simulink model "detector"  (R2018b)
settings: Solver=FixedStepDiscrete  StartTime=0.0  StopTime=10.0  RelTol=1e-3
libraries: hdlsllib x18, simulink x18
settings Model: Creator=jayakumarav  LastModifiedBy=hiterd
settings DebuggingCC: LibraryContextMissingDiagnostic=none
settings SFSimCC: SimUseLocalCustomCode=off
settings RTWCC: RTWUseLocalCustomCode=off

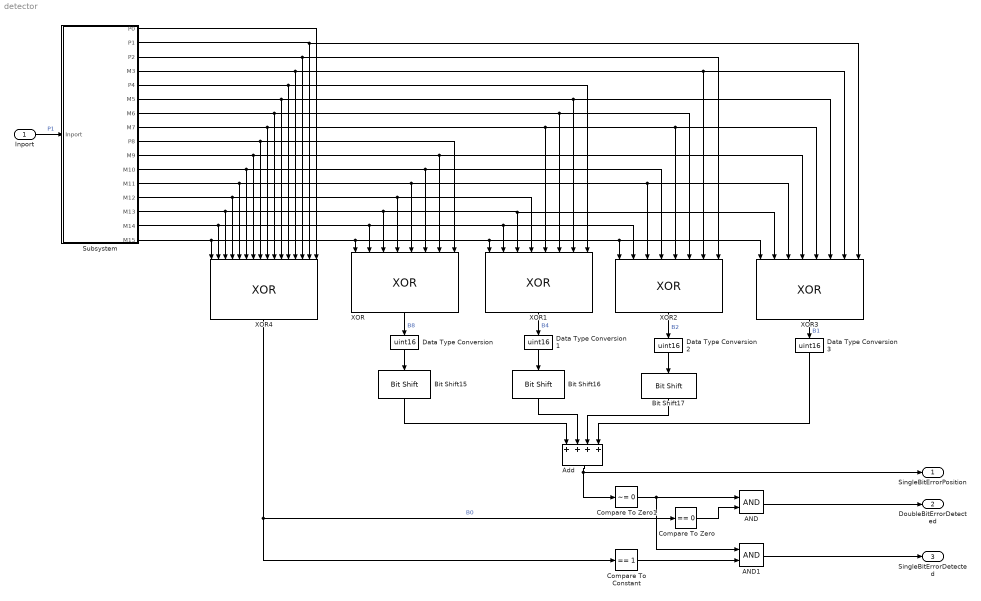
== system detector ==
  Inport : Inport
  AND : Logic  AllPortsSameDT=off  OutDataTypeStr=boolean
  AND1 : Logic  AllPortsSameDT=off  OutDataTypeStr=boolean
  Add : Sum  Inputs=++++
  Bit Shift15 : hdlsllib/Logic and Bit Operations/Bit Shift  mode=Shift Left Logical  N=3
      settings: SourceProductName=HDL Coder  SourceProductBaseCode=HD
  Bit Shift16 : hdlsllib/Logic and Bit Operations/Bit Shift  mode=Shift Left Logical  N=2
      settings: SourceProductName=HDL Coder  SourceProductBaseCode=HD
  Bit Shift17 : hdlsllib/Logic and Bit Operations/Bit Shift  mode=Shift Left Logical  N=1
      settings: SourceProductName=HDL Coder  SourceProductBaseCode=HD
  Compare To Constant : simulink/Logic and Bit Operations/Compare To Constant  relop===  const=1  OutDataTypeStr=boolean
  Compare To Zero : simulink/Logic and Bit Operations/Compare To Zero  relop===  OutDataTypeStr=boolean
  Compare To Zero1 : simulink/Logic and Bit Operations/Compare To Zero  relop=~=  OutDataTypeStr=boolean
  Data Type Conversion{,1..3} (4 alike) : DataTypeConversion  OutDataTypeStr=uint16
  Subsystem : Subsystem
  XOR{,1..3} (4 alike) : Logic  Operator=XOR  Inputs=8  IconShape=distinctive  AllPortsSameDT=off  OutDataTypeStr=boolean
  XOR4 : Logic  Operator=XOR  Inputs=16  IconShape=distinctive  AllPortsSameDT=off  OutDataTypeStr=boolean
  SingleBitErrorPosition : Outport
  DoubleBitErrorDetected : Outport  Port=2
  SingleBitErrorDetected : Outport  Port=3
  wires:
  Subsystem/9(P8) -> XOR/8, XOR4/8
  XOR/1 -> Data Type Conversion/1  "B8"
  Subsystem/14(M13) -> XOR3/2, XOR1/3, XOR/3, XOR4/3
  Subsystem/10(M9) -> XOR3/4, XOR/7, XOR4/7
  Subsystem/4(M3) -> XOR4/13, XOR3/7, XOR2/7
  Compare To Constant/1 -> AND1/2
  Bit Shift15/1 -> Add/1
  Bit Shift16/1 -> Add/2
  Subsystem/12(M11) -> XOR2/3, XOR3/3, XOR/5, XOR4/5
  Subsystem/2(P1) -> XOR3/8, XOR4/15
  Subsystem/11(M10) -> XOR2/4, XOR/6, XOR4/6
  Subsystem/1(P0) -> XOR4/16
  Subsystem/16(M15) -> XOR2/1, XOR3/1, XOR1/1, XOR/1, XOR4/1
  Data Type Conversion1/1 -> Bit Shift16/1
  AND1/1 -> SingleBitErrorDetected/1
  Subsystem/5(P4) -> XOR1/8, XOR4/12
  Data Type Conversion3/1 -> Add/4
  Compare To Zero/1 -> AND/2
  AND/1 -> DoubleBitErrorDetected/1
  Compare To Zero1/1 -> AND/1, AND1/1
  Add/1 -> Compare To Zero1/1, SingleBitErrorPosition/1
  XOR2/1 -> Data Type Conversion2/1  "B2"
  XOR3/1 -> Data Type Conversion3/1  "B1"
  Data Type Conversion/1 -> Bit Shift15/1
  XOR4/1 -> Compare To Constant/1, Compare To Zero/1  "B0"
  Subsystem/6(M5) -> XOR3/6, XOR1/7, XOR4/11
  Inport/1 -> Subsystem/1(Inport)  "P1"
  Subsystem/7(M6) -> XOR1/6, XOR2/6, XOR4/10
  Subsystem/3(P2) -> XOR2/8, XOR4/14
  Subsystem/15(M14) -> XOR1/2, XOR2/2, XOR/2, XOR4/2
  Bit Shift17/1 -> Add/3
  Subsystem/13(M12) -> XOR1/4, XOR/4, XOR4/4
  Data Type Conversion2/1 -> Bit Shift17/1
  XOR1/1 -> Data Type Conversion1/1  "B4"
  Subsystem/8(M7) -> XOR3/5, XOR2/5, XOR1/5, XOR4/9

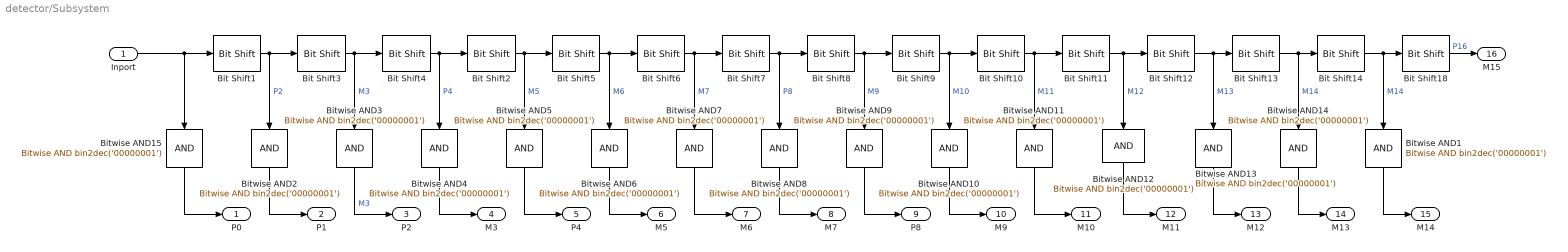
== system detector/Subsystem ==
  Inport : Inport  OutDataTypeStr=uint16
  Bit Shift{1..14,18} (15 alike) : hdlsllib/Logic and Bit Operations/Bit Shift  mode=Shift Right Logical  N=1
      settings: SourceProductName=HDL Coder  SourceProductBaseCode=HD
  Bitwise AND{1..15} (15 alike) : simulink/Logic and Bit Operations/Bitwise Operator  logicop=AND  UseBitMask=on  BitMask=bin2dec('00000001')  BitMaskRealWorld=Stored Integer
  P0 : Outport
  P1 : Outport  Port=2
  P2 : Outport  Port=3
  M3 : Outport  Port=4
  P4 : Outport  Port=5
  M5 : Outport  Port=6
  M6 : Outport  Port=7
  M7 : Outport  Port=8
  P8 : Outport  Port=9
  M9 : Outport  Port=10
  M10 : Outport  Port=11
  M11 : Outport  Port=12
  M12 : Outport  Port=13
  M13 : Outport  Port=14
  M14 : Outport  Port=15
  M15 : Outport  Port=16
  wires:
  Bit Shift8/1 -> Bit Shift9/1, Bitwise AND9/1  "M9"
  Bit Shift10/1 -> Bit Shift11/1, Bitwise AND11/1  "M11"
  Bit Shift11/1 -> Bit Shift12/1, Bitwise AND12/1  "M12"
  Bitwise AND3/1 -> P2/1  "M3"
  Bit Shift6/1 -> Bit Shift7/1, Bitwise AND7/1  "M7"
  Bitwise AND9/1 -> P8/1
  Bit Shift3/1 -> Bit Shift4/1, Bitwise AND3/1  "M3"
  Bitwise AND7/1 -> M6/1
  Bit Shift12/1 -> Bitwise AND13/1, Bit Shift13/1  "M13"
  Bit Shift2/1 -> Bit Shift5/1, Bitwise AND5/1  "M5"
  Bitwise AND5/1 -> P4/1
  Bit Shift1/1 -> Bit Shift3/1, Bitwise AND2/1  "P2"
  Bitwise AND12/1 -> M11/1
  Bitwise AND13/1 -> M12/1
  Bit Shift18/1 -> M15/1  "P16"
  Bit Shift4/1 -> Bit Shift2/1, Bitwise AND4/1  "P4"
  Bit Shift5/1 -> Bit Shift6/1, Bitwise AND6/1  "M6"
  Bit Shift9/1 -> Bit Shift10/1, Bitwise AND10/1  "M10"
  Bitwise AND6/1 -> M5/1
  Bit Shift7/1 -> Bit Shift8/1, Bitwise AND8/1  "P8"
  Bit Shift13/1 -> Bitwise AND14/1, Bit Shift14/1  "M14"
  Bitwise AND8/1 -> M7/1
  Inport/1 -> Bitwise AND15/1, Bit Shift1/1
  Bitwise AND11/1 -> M10/1
  Bitwise AND4/1 -> M3/1
  Bitwise AND10/1 -> M9/1
  Bitwise AND14/1 -> M13/1
  Bitwise AND2/1 -> P1/1
  Bit Shift14/1 -> Bitwise AND1/1, Bit Shift18/1  "M14"
  Bitwise AND1/1 -> M14/1
  Bitwise AND15/1 -> P0/1
